simulink model "task2"  (R2021b)
settings: Solver=FixedStepAuto  StartTime=0.0  StopTime=10.0  RelTol=1e-3
libraries: dspfdesign x2, commdigbbndam3 x2, commchan3 x1, commrandsrc3 x1, commfilt2 x1
settings Model: Creator=ksksks  LastModifiedBy=ksksks

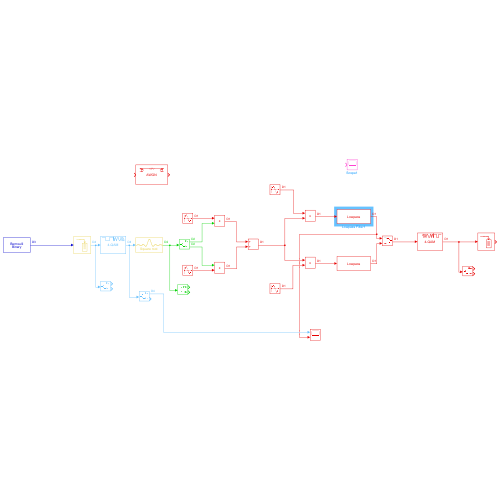
[thumbnail: Simulink's stored preview of the top-level diagram]
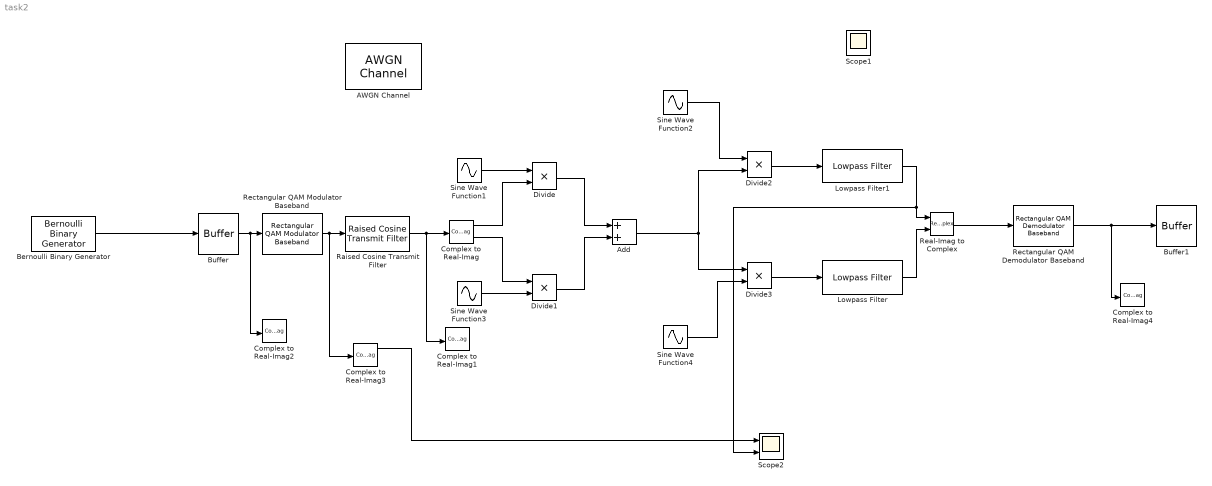
== system task2 ==
  AWGN Channel : commchan3/AWGN Channel  InputProcessing=Columns as channels (frame based)  seed=67  noiseMode="Signal to noise ratio  (Eb/No)"  EbNodB=10  EsNodB=10  SNRdB=10  bitsPerSym=1  Ps=1  Tsym=1  variance=1
  Add : Sum
  Bernoulli Binary Generator : commrandsrc3/Bernoulli Binary Generator  ProbabilityOfZero=0.5  SeedSource=Auto  Seed=0  SampleTime=1e-6  SamplesPerFrame=1  OutputDataType=double  SimulateUsing=Interpreted execution
  Buffer : Buffer  N=2  OutputFrames=off
  Buffer1 : Buffer  N=2  OutputFrames=off
  Complex to Real-Imag{,1..4} (5 alike) : ComplexToRealImag
  Divide{,1..3} (4 alike) : Product  Inputs=**
  Lowpass Filter : dspfdesign/Lowpass Filter  FilterType=FIR  DesignForMinimumOrder=off  FilterOrder=20  PassbandFrequency=1e6  StopbandFrequency=3e-6  PassbandRipple=2  StopbandAttenuation=60  InheritSampleRate=off  SampleRate=1e8  SimulateUsing=Interpreted execution  roundingMode=Floor  coeffsDataTypeStr=fixdt(1,16)
  Lowpass Filter1 : dspfdesign/Lowpass Filter  FilterType=FIR  DesignForMinimumOrder=off  FilterOrder=20  PassbandFrequency=1e6  StopbandFrequency=3e-6  PassbandRipple=2  StopbandAttenuation=60  InheritSampleRate=off  SampleRate=1e8  SimulateUsing=Interpreted execution  roundingMode=Floor  coeffsDataTypeStr=fixdt(1,16)
  Raised Cosine Transmit Filter : commfilt2/Raised Cosine Transmit Filter  filtType=Square root  R=0.8  filtSpan=4  N=8  filterGain=1  RateOptions=Allow multirate processing  framing=Mute  checkCoeff=off  variableName=rcTxFilt  checkGain=Normalized  sampMode=Mute  saveAsFlag=0  currentFiltSpan=10  D=5  launchFVT=on  roundingMode=Floor  overflowMode=off  coeffDataTypeStr=Inherit: Same word length as input  coeffMin=[]  coeffMax=[]  coeffLastDataTypeStr=Inherit: Same word length as input  outputDataTypeStr=Inherit: Same as accumulator  outputMin=[]  outputMax=[]  outputLastDataTypeStr=Inherit: Same as accumulator
  Real-Imag to Complex : RealImagToComplex
  Rectangular QAM Demodulator Baseband : commdigbbndam3/Rectangular QAM Demodulator Baseband  M=4  OutType=Bit  DecType=Hard decision  VarSource=Dialog  Variance=1  Dec=Gray  Mapping=[0:15]  PowType=Min. distance between symbols  MinDist=20000000  AvgPow=1  PeakPow=1  Ph=pi/4  outDtype1=Inherit via internal rule  outDtype2=Inherit via internal rule  derotateFactorWordLen=16  derotateFactorDataTypeStr=Inherit: Same word length as input  derotateFactorLastDataTypeStr=Inherit: Same word length as input  denormFactorWordLen=16  denormFactorDataTypeStr=Inherit: Same word length as input  denormFactorLastDataTypeStr=Inherit: Same word length as input  prodOutWordLen=32  prodOutOverflowMode=Wrap  prodOutRoundingMode=Floor  prodOutOvFlMode=off  prodOutOvFlModeLastStrValue=off  sumWordLen=32
  Rectangular QAM Modulator Baseband : commdigbbndam3/Rectangular QAM Modulator Baseband  M=4  InType=Bit  Enc=Gray  Mapping=[0:15]  PowType=Min. distance between symbols  MinDist=2  AvgPow=1  PeakPow=1  Ph=pi/4  outDtype=double  outWordLen=16  outUDDataType=sfix(16)  outFracLenMode=Best precision  outFracLen=15  outDataTypeStr=double  outLastDataTypeStr=double
  Scope1 : Scope
  Scope2 : Scope  NumInputPorts=2
  Sine Wave Function{1..4} (4 alike) : Sin  SineType=Sample based  Frequency=1e-8  Samples=20  SampleTime=1e-8
  wires:
  Bernoulli Binary Generator/1 -> Buffer/1
  Buffer/1 -> Complex to Real-Imag2/1, Rectangular QAM Modulator Baseband/1
  Complex to Real-Imag/1 -> Divide/2
  Complex to Real-Imag/2 -> Divide1/1
  Sine Wave Function3/1 -> Divide1/2
  Sine Wave Function1/1 -> Divide/1
  Divide/1 -> Add/1
  Divide1/1 -> Add/2
  Rectangular QAM Modulator Baseband/1 -> Complex to Real-Imag3/1, Raised Cosine Transmit Filter/1
  Raised Cosine Transmit Filter/1 -> Complex to Real-Imag1/1, Complex to Real-Imag/1
  Add/1 -> Divide3/1, Divide2/2
  Sine Wave Function2/1 -> Divide2/1
  Sine Wave Function4/1 -> Divide3/2
  Divide3/1 -> Lowpass Filter/1
  Divide2/1 -> Lowpass Filter1/1
  Lowpass Filter1/1 -> Scope2/2, Real-Imag to Complex/1
  Lowpass Filter/1 -> Real-Imag to Complex/2
  Real-Imag to Complex/1 -> Rectangular QAM Demodulator Baseband/1
  Rectangular QAM Demodulator Baseband/1 -> Complex to Real-Imag4/1, Buffer1/1
  Complex to Real-Imag3/1 -> Scope2/1
